simulink model "kps6_T"  (R2020a)
settings: Solver=VariableStepAuto  StartTime=0.0  StopTime=1000  RelTol=1e-3
libraries: simulink x6, roblocks x1
settings Model: EnablePacing=on  Creator=hemingshan  LastModifiedBy=hemingshan

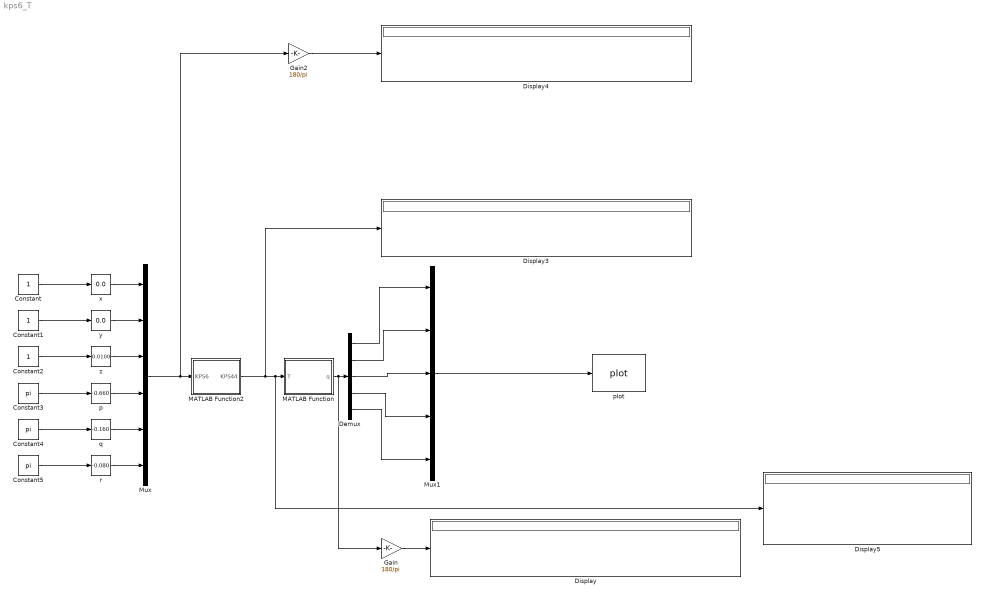
== system kps6_T ==
  Constant : Constant
  Constant1 : Constant
  Constant2 : Constant
  Constant3 : Constant  Value=pi
  Constant4 : Constant  Value=pi
  Constant5 : Constant  Value=pi
  Demux : Demux  Outputs=5
  Display{,3..5} (4 alike) : Display
  Gain : Gain  Gain=180/pi
  Gain2 : Gain  Gain=180/pi
  MATLAB Function : MATLAB Function  TreatAsAtomicUnit=on
  MATLAB Function2 : MATLAB Function  TreatAsAtomicUnit=on
  Mux : Mux  Inputs=6
  Mux1 : Mux  Inputs=5
  p : simulink/Math Operations/Slider Gain  gain=-0.660  low=-1  high=1
  plot : roblocks/Arm/plot  robot=robot  fps=5  holdplot=on
  q : simulink/Math Operations/Slider Gain  gain=-0.160  low=-1  high=1
  r : simulink/Math Operations/Slider Gain  gain=-0.080  low=-1  high=1
  x : simulink/Math Operations/Slider Gain  gain=0.0  low=-2  high=2
  y : simulink/Math Operations/Slider Gain  gain=0.0  low=-1  high=1
  z : simulink/Math Operations/Slider Gain  gain=0.0100  low=-10  high=1
  wires:
  Gain2/1 -> Display4/1
  Constant3/1 -> p/1
  Demux/3 -> Mux1/3
  Demux/4 -> Mux1/4
  Constant/1 -> x/1
  Mux1/1 -> plot/1
  Mux/1 -> Gain2/1, MATLAB Function2/1(KPS6)
  Constant1/1 -> y/1
  Demux/5 -> Mux1/5
  q/1 -> Mux/5
  MATLAB Function/1(q) -> Demux/1, Gain/1
  Demux/2 -> Mux1/2
  Gain/1 -> Display/1
  MATLAB Function2/1(KPS44) -> Display3/1, Display5/1, MATLAB Function/1(T)
  Constant2/1 -> z/1
  p/1 -> Mux/4
  x/1 -> Mux/1
  Constant4/1 -> q/1
  y/1 -> Mux/2
  Demux/1 -> Mux1/1
  z/1 -> Mux/3
  Constant5/1 -> r/1
  r/1 -> Mux/6

== matlab function kps6_T/MATLAB Function2 ==
  data: KPS6 input; KPS44 output
function KPS44  = IK(KPS6)
%% input 
x = KPS6(1);
y = KPS6(2);
z = KPS6(3);
p = KPS6(4);
q = KPS6(5);
r = KPS6(6);
%% output
I= zeros(4,4);
%%
sx = sin(p);
cx = cos(p);
sy = sin(q);
cy = cos(q);
sz = sin(r);
cz = cos(r);
I(1,1) = cy*cz; I(1,2) = cz*sx*sy-cx*sz; I(1,3) =sx*sz+cx*cz*sy;
I(2,1) = cy*sz; I(2,2) = cx*cz+sx*sy*sz; I(2,3) =cx*sy*sz-cz*sx;
I(3,1) = -sy; I(3,2) = cy*sx; I(3,3) = cx*cy;
% I(1,1) = 1; I(1,2) = 0; I(1,3) =0;
% I(2,1) = 0; I(2,2) = 1; I(2,3) =0;
% I(3,1) = 0; I(3,2) = 0; I(3,3) =1;
I(1,4)=x+0.06428;I(2,4)=y;I(3,4)=z-0.5273;I(4,4)=1;
%%
KPS44 = I;
end

== matlab function kps6_T/MATLAB Function ==
  data: T input; q output
function q= fcn(T)
%theta-offset
% offset1 = 0;
% offset2 = pi/2-atan(0.23966/0.28189);
% offset3 = pi/2-atan(0.23966/0.28189)+atan(0.15989/0.31135);
% offset4 = -atan(0.15989/0.31135);
%%DH
d1 = -0.097;
a3 = -sqrt(0.23966^2+0.28189^2);
a4 = -sqrt(-0.15989^2+0.31135^2);
%%theta1
  theta1 = atan2(T(2,4),T(1,4));
  if theta1 > pi/2
      theta1 = pi - theta1;
  end
%%theta3
  equ1 = T(1,4)^2 + T(2,4)^2;
  equ2 = (T(3,4)-d1)^2;
  equ3 = equ1 + equ2;
  c3   = (equ3 - a3^2 - a4^2)/(2*a3*a4);
%   s3   = sqrt(1-c3^2);
  if 1-c3^2 < 1e-20
      s3 = 0;
  else
      s3   = sqrt(1-c3^2);
  end
  theta3 = atan2(s3,c3);
  
%%theta2
  
  x = (T(1,4)^2+T(2,4)^2)^0.5;
  y = T(3,4)-d1;
  if T(1,4) < 0
      x = -x;
  end
  k1 = (a4*cos(theta3)+a3);
  k2 = -sin(theta3)*a4;
  theta2 = atan2(y,x)+ atan2(k2,k1);
  
%   atan = atan2(k2,k1)
%   theta2 = -theta2;
  
%%theta4
  phi = atan2(T(3,1),T(3,2));
  theta4 = phi - theta2 - theta3;
  q = [0,theta1,theta2,theta3,theta4];
